simulink model "adcs_sim_main"  (R2016b)
settings: Solver=VariableStepAuto  StartTime=0.0  StopTime=360  RelTol=1e-3  EnableMultiTasking=on
InitFcn:
  | %sim_init
StopFcn:
  | %% Extract States
  | %states = logsout.getElement('states').Values;
  | %sc_quat = states.quaternion;
  | %omega_radps = states.body_rates_radps;
  | %pos_eci_km = states.position_eci_km;
  | %vel_eci_kmps = states.velocity_eci_kmps;
  | 
  | %% Extract Actuator measurements
  | %act_meas = logsout.getElement('act_meas').Values;
  | 
  | %% Extract Commands
  | %cmds = logsout.getElement('commands').Values;
  | %MT_dv = cmds.MT_dv;
  | 
  | %% Extract B-dot tumble status
  | %tumble = logsout.getElement('tumble').Values;
  | %tumble_t = logsout.getElement('tumble').Time;
undefined symbols (not defined in the file): adcs_fsw_main, CAN, CAN_lib, cmd_MT_fsw_dv, env_estimation_lib, Flightsoftware, fsw_params, MET, MSP_FSW, MSP_FSW_lib, orbit_TLE, sc_mode, sim_params
libraries: bus_stubs_fsw x2, actuators_lib x1, dynamics_lib x1, environment_lib x1, MET_lib x1, MSP_BDOT_lib x1, CAN_out_lib x1, extended_kalman_filter_lib x1, actuator_processing x1, command_generation x1, time_conversion_lib x1, gs_prediction_lib x1
settings Model: Creator=bbarz_000  LastModifiedBy=taylorreynolds
settings DataIOCC: SaveOutput=off
settings OptimizationCC: DefaultParameterBehavior=Inlined  UseDivisionForNetSlopeComputation=on  UseFloatMulNetSlope=on  InlineInvariantSignals=on  PassReuseOutputArgsAs=Individual arguments  ZeroExternalMemoryAtStartup=off  ZeroInternalMemoryAtStartup=off  NoFixptDivByZeroProtection=on  EfficientFloat2IntCast=on  LifeSpan=1
settings DebuggingCC: ParameterTunabilityLossMsg=error  SFUnexpectedBacktrackingDiag=warning  SFNoUnconditionalDefaultTransitionDiag=warning  SFExecutionAtInitializationDiag=none
settings HardwareCC: ProdBitPerInt=16  ProdBitPerPointer=16  ProdBitPerSizeT=16  ProdBitPerPtrDiffT=16  ProdLargestAtomicFloat=None  ProdWordSize=16  ProdHWDeviceType=Texas Instruments->MSP430
settings RTWCC: SystemTargetFile=ert.tlc  GenCodeOnly=on  PackageGeneratedCodeAndArtifacts=on  TemplateMakefile=ert_default_tmf  Description=Embedded Coder  GenerateReport=on  Toolchain=Clang v3.1 | gmake (64-bit Mac)  IncludeHyperlinkInReport=on  LaunchReport=on  GenerateTraceInfo=on  GenerateTraceReport=on  GenerateTraceReportSl=on  GenerateTraceReportSf=on  GenerateTraceReportEml=on  GenerateCodeMetricsReport=on
settings CodeAppCC: ForceParamTrailComments=on  IgnoreCustomStorageClasses=off  OperatorAnnotations=on  SimulinkDataObjDesc=on  SFDataObjDesc=on  MATLABFcnDesc=on  CustomSymbolStrGlobalVar=rt$N$M  CustomSymbolStrType=$N$M  CustomSymbolStrFcn=$N$M$F  CustomSymbolStrMacro=$N$M  InsertBlockDesc=on  MATLABSourceComments=on
settings ERTTargetCC: GenerateSampleERTMain=on  CombineSignalStateStructs=on  SupportComplex=off  SupportContinuousTime=on  SupportNonInlinedSFcns=on  InlinedParameterPlacement=NonHierarchical  ERTCustomFileTemplate=example_file_process.tlc  ERTFilePackagingFormat=CompactWithDataFile
settings ConfigComp: CovMetricSettings=dw  CovHtmlReporting=on  CovSaveCumulativeToWorkspaceVar=on  CovSaveSingleToWorkspaceVar=on  CovExternalEMLEnable=off

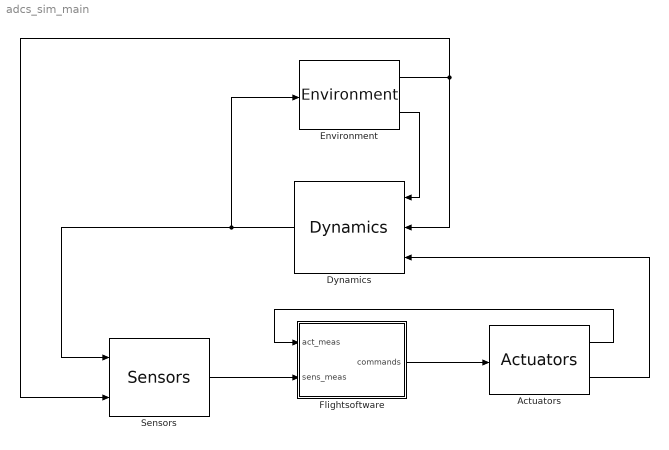
== system adcs_sim_main ==
  Actuators : actuators_lib/Actuators
  Dynamics : dynamics_lib/Dynamics
  Environment : environment_lib/Environment
  Flightsoftware : Subsystem  AncestorBlock=adcs_fsw_main/Flightsoftware
  Sensors : sensors_lib/Sensors
  wires:
  Flightsoftware/1(commands) -> Actuators/1
  Dynamics/1 -> Environment/1, Sensors/1
  Sensors/1 -> Flightsoftware/2(sens_meas)
  Environment/1 -> Sensors/2, Dynamics/2
  Actuators/2 -> Dynamics/3
  Actuators/1 -> Flightsoftware/1(act_meas)
  Environment/2 -> Dynamics/1

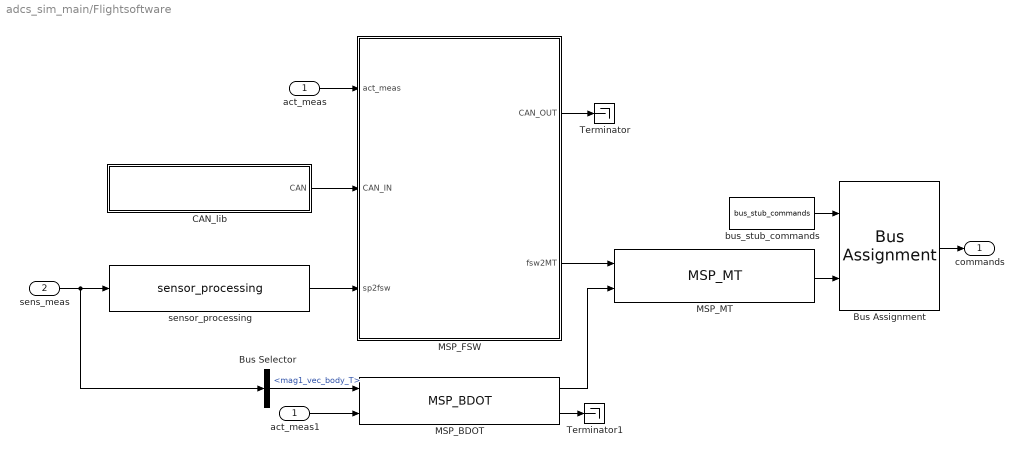
== system adcs_sim_main/Flightsoftware ==
  act_meas : Inport  OutDataTypeStr=Bus: act_meas
  sens_meas : Inport  Port=2  OutDataTypeStr=Bus: sens_meas
  Bus Assignment : BusAssignment  AssignedSignals=MT_dv
  Bus Selector : BusSelector  OutputSignals=mag1_vec_body_T
  CAN_lib : Subsystem  AncestorBlock=CAN_lib/CAN_lib
  MSP_BDOT : MSP_BDOT_lib/MSP_BDOT
  MSP_FSW : Subsystem  AncestorBlock=MSP_FSW_lib/MSP_FSW
  MSP_MT : MSP_MT_lib/MSP_MT
  Terminator : Terminator
  Terminator1 : Terminator
  act_meas1 : InportShadow  OutDataTypeStr=Bus: act_meas
  bus_stub_commands : bus_stubs_template/bus_stub_commands
  sensor_processing : sensor_processing/sensor_processing
  commands : Outport
  wires:
  act_meas1/1 -> MSP_BDOT/2
  MSP_BDOT/2 -> Terminator1/1
  MSP_FSW/1(CAN_OUT) -> Terminator/1
  CAN_lib/1(CAN) -> MSP_FSW/2(CAN_IN)
  act_meas/1 -> MSP_FSW/1(act_meas)
  sensor_processing/1 -> MSP_FSW/3(sp2fsw)
  MSP_FSW/2(fsw2MT) -> MSP_MT/1
  MSP_BDOT/1 -> MSP_MT/2
  MSP_MT/1 -> Bus Assignment/2
  Bus Selector/1 -> MSP_BDOT/1  "<mag1_vec_body_T>"
  sens_meas/1 -> Bus Selector/1, sensor_processing/1
  bus_stub_commands/1 -> Bus Assignment/1
  Bus Assignment/1 -> commands/1

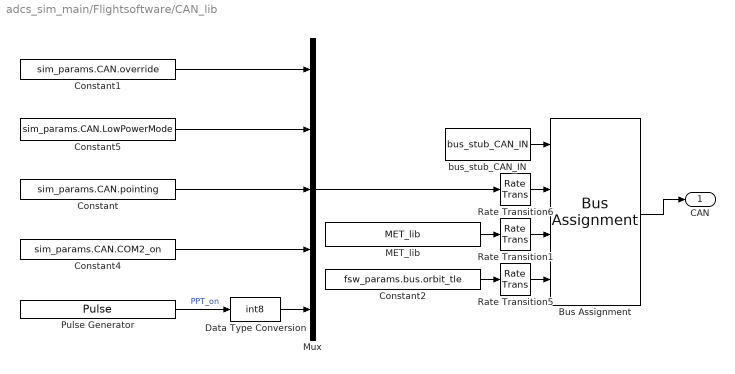
== system adcs_sim_main/Flightsoftware/CAN_lib ==
  Bus Assignment : BusAssignment  AssignedSignals=CAN,MET,orbit_TLE
  Constant : Constant  Value=sim_params.CAN.pointing  OutDataTypeStr=int8
  Constant1 : Constant  Value=sim_params.CAN.override  OutDataTypeStr=int8
  Constant2 : Constant  Value=fsw_params.bus.orbit_tle
  Constant4 : Constant  Value=sim_params.CAN.COM2_on  OutDataTypeStr=int8
  Constant5 : Constant  Value=sim_params.CAN.LowPowerMode  OutDataTypeStr=int8
  Data Type Conversion : DataTypeConversion  OutDataTypeStr=int8
  MET_lib : MET_lib/MET_lib
  Mux : Mux  Inputs=5
  Pulse Generator : DiscretePulseGenerator  PulseType=Time based  Period=sim_params.CAN.sync_pulse_period_s  PulseWidth=sim_params.CAN.PPT_on_sync_pct
  Rate Transition1 : RateTransition  X0=sim_params.CAN.ic.MET  OutPortSampleTime=sim_params.CAN.sample_time_s
  Rate Transition5 : RateTransition  X0=fsw_params.bus.orbit_tle  OutPortSampleTime=sim_params.CAN.sample_time_s
  Rate Transition6 : RateTransition  X0=sim_params.CAN.ic.all  OutPortSampleTime=sim_params.CAN.sample_time_s
  bus_stub_CAN_IN : bus_stubs_fsw/bus_stub_CAN_IN
  CAN : Outport
  wires:
  Data Type Conversion/1 -> Mux/5
  Rate Transition1/1 -> Bus Assignment/3
  Rate Transition6/1 -> Bus Assignment/2
  Rate Transition5/1 -> Bus Assignment/4
  Constant2/1 -> Rate Transition5/1
  MET_lib/1 -> Rate Transition1/1
  Pulse Generator/1 -> Data Type Conversion/1  "PPT_on"
  Constant4/1 -> Mux/4
  Constant/1 -> Mux/3
  Constant5/1 -> Mux/2
  Constant1/1 -> Mux/1
  Mux/1 -> Rate Transition6/1
  bus_stub_CAN_IN/1 -> Bus Assignment/1
  Bus Assignment/1 -> CAN/1

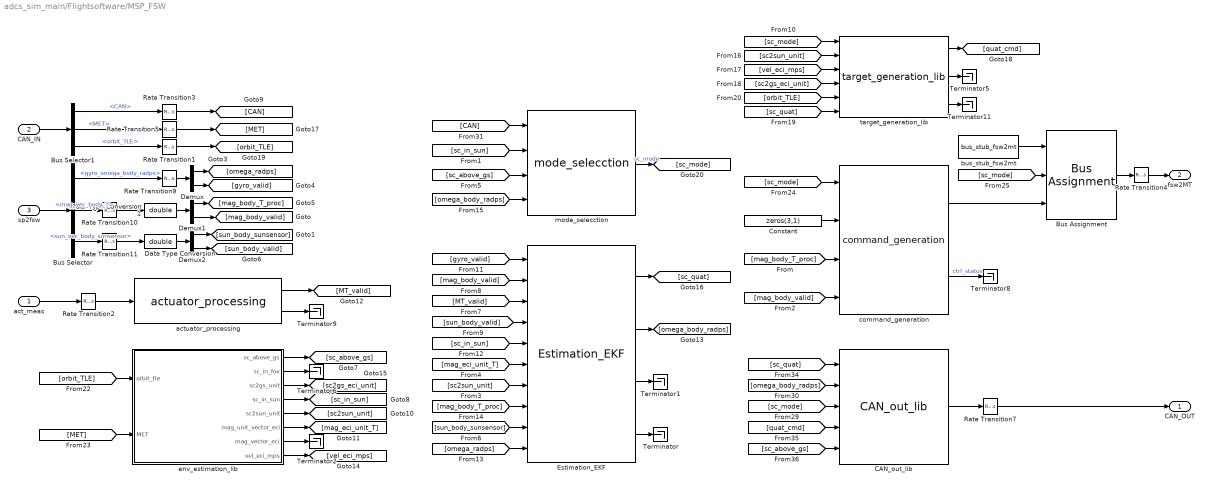
== system adcs_sim_main/Flightsoftware/MSP_FSW ==
  act_meas : Inport
  CAN_IN : Inport  Port=2  OutDataTypeStr=Bus: CAN_IN
  sp2fsw : Inport  Port=3  OutDataTypeStr=Bus: sp2fsw
  Bus Assignment : BusAssignment  AssignedSignals=sc_mode,cmd_MT_fsw_dv
  Bus Selector : BusSelector  OutputSignals=gyro_omega_body_radps,mag_vec_body_T,sun_vec_body_sunsensor
  Bus Selector1 : BusSelector  OutputSignals=CAN,MET,orbit_TLE
  CAN_out_lib : CAN_out_lib/CAN_out_lib
  Constant : Constant  Value=zeros(3,1)
  Data Type Conversion : DataTypeConversion  OutDataTypeStr=double
  Data Type Conversion1 : DataTypeConversion  OutDataTypeStr=double
  Demux : Demux  Outputs=[3 1]
  Demux1 : Demux  Outputs=[3 1]
  Demux2 : Demux  Outputs=[3 1]
  "Estimation_EKF " : extended_kalman_filter_lib/Estimation_EKF 
  Rate Transition1 : RateTransition  X0=fsw_params.bus.orbit_tle  OutPortSampleTime=fsw_params.sample_time_s
  Rate Transition{2,9..11} (4 alike) : RateTransition  OutPortSampleTime=fsw_params.sample_time_s
  Rate Transition3 : RateTransition  X0=fsw_params.bus.CAN_ic  OutPortSampleTime=fsw_params.sample_time_s
  Rate Transition4 : RateTransition
  Rate Transition5 : RateTransition  X0=fsw_params.bus.MET_epoch  OutPortSampleTime=fsw_params.sample_time_s
  Rate Transition7 : RateTransition
  Terminator{,1..2,5..6,8..9,11} (8 alike) : Terminator
  actuator_processing : actuator_processing/actuator_processing
  bus_stub_fsw2mt : bus_stubs_fsw/bus_stub_fsw2mt
  command_generation : command_generation/command_generation
  env_estimation_lib : Subsystem  AncestorBlock=env_estimation_lib/env_estimation_lib
  mode_selecction : mode_selection/mode_selecction
  target_generation_lib : target_generation_lib/target_generation_lib
  CAN_OUT : Outport
  fsw2MT : Outport  Port=2
  wires:
  Data Type Conversion1/1 -> Demux1/1
  Data Type Conversion/1 -> Demux2/1
  Demux1/2 -> [mag_body_valid]
  Demux1/1 -> [mag_body_T_proc]
  Bus Selector1/2 -> Rate Transition5/1  "<MET>"
  Rate Transition5/1 -> [MET]
  [sc_mode] -> Bus Assignment/2
  [sc_mode] -> command_generation/1
  [sc_mode] -> target_generation_lib/1
  mode_selecction/1 -> [sc_mode]  "sc_mode"
  [MET] -> env_estimation_lib/2(MET)
  [orbit_TLE] -> env_estimation_lib/1(orbit_tle)
  Bus Selector1/3 -> Rate Transition1/1  "<orbit_TLE>"
  Rate Transition1/1 -> [orbit_TLE]
  Constant/1 -> command_generation/2
  command_generation/1 -> Bus Assignment/3
  [mag_body_T_proc] -> command_generation/3
  [quat_cmd] -> CAN_out_lib/4
  target_generation_lib/3 -> Terminator11/1
  [sc_above_gs] -> CAN_out_lib/5
  [sc_quat] -> CAN_out_lib/1
  [omega_body_radps] -> CAN_out_lib/2
  [sc_mode] -> CAN_out_lib/3
  [CAN] -> mode_selecction/1
  Rate Transition7/1 -> CAN_OUT/1
  Rate Transition4/1 -> fsw2MT/1
  CAN_IN/1 -> Bus Selector1/1
  Rate Transition2/1 -> actuator_processing/1
  sp2fsw/1 -> Bus Selector/1
  CAN_out_lib/1 -> Rate Transition7/1
  Bus Assignment/1 -> Rate Transition4/1
  bus_stub_fsw2mt/1 -> Bus Assignment/1
  target_generation_lib/2 -> Terminator5/1
  target_generation_lib/1 -> [quat_cmd]
  [orbit_TLE] -> target_generation_lib/5
  [sc_quat] -> target_generation_lib/6
  [sc2gs_eci_unit] -> target_generation_lib/4
  [vel_eci_mps] -> target_generation_lib/3
  [sc2sun_unit] -> target_generation_lib/2
  [omega_body_radps] -> mode_selecction/4
  "Estimation_EKF "/2 -> [omega_body_radps]
  actuator_processing/2 -> Terminator9/1
  actuator_processing/1 -> [MT_valid]
  act_meas/1 -> Rate Transition2/1
  Demux2/2 -> [sun_body_valid]
  Demux2/1 -> [sun_body_sunsensor]
  Bus Selector/3 -> Rate Transition11/1  "<sun_vec_body_sunsensor>"
  Rate Transition10/1 -> Data Type Conversion1/1
  Bus Selector/2 -> Rate Transition10/1  "<mag_vec_body_T>"
  Demux/2 -> [gyro_valid]
  Demux/1 -> [omega_radps]
  Bus Selector/1 -> Rate Transition9/1  "<gyro_omega_body_radps>"
  [sc_in_sun] -> mode_selecction/2
  [mag_body_valid] -> "Estimation_EKF "/2
  [gyro_valid] -> "Estimation_EKF "/1
  env_estimation_lib/4(sc_in_sun) -> [sc_in_sun]
  [MT_valid] -> "Estimation_EKF "/3
  [sun_body_valid] -> "Estimation_EKF "/4
  [sc_in_sun] -> "Estimation_EKF "/5
  "Estimation_EKF "/4 -> Terminator/1
  "Estimation_EKF "/3 -> Terminator1/1
  env_estimation_lib/5(sc2sun_unit) -> [sc2sun_unit]
  env_estimation_lib/6(mag_unit_vector_eci) -> [mag_eci_unit_T]
  env_estimation_lib/7(mag_vector_eci) -> Terminator2/1
  env_estimation_lib/8(vel_eci_mps) -> [vel_eci_mps]
  env_estimation_lib/2(sc_in_fov) -> Terminator6/1
  env_estimation_lib/3(sc2gs_unit) -> [sc2gs_eci_unit]
  [omega_radps] -> "Estimation_EKF "/10
  [sun_body_sunsensor] -> "Estimation_EKF "/9
  [mag_body_T_proc] -> "Estimation_EKF "/8
  [mag_eci_unit_T] -> "Estimation_EKF "/6
  [sc2sun_unit] -> "Estimation_EKF "/7
  [mag_body_valid] -> command_generation/4
  command_generation/2 -> Terminator8/1  "ctrl_status"
  "Estimation_EKF "/1 -> [sc_quat]
  env_estimation_lib/1(sc_above_gs) -> [sc_above_gs]
  [sc_above_gs] -> mode_selecction/3
  Rate Transition9/1 -> Demux/1
  Rate Transition11/1 -> Data Type Conversion/1
  Bus Selector1/1 -> Rate Transition3/1  "<CAN>"
  Rate Transition3/1 -> [CAN]

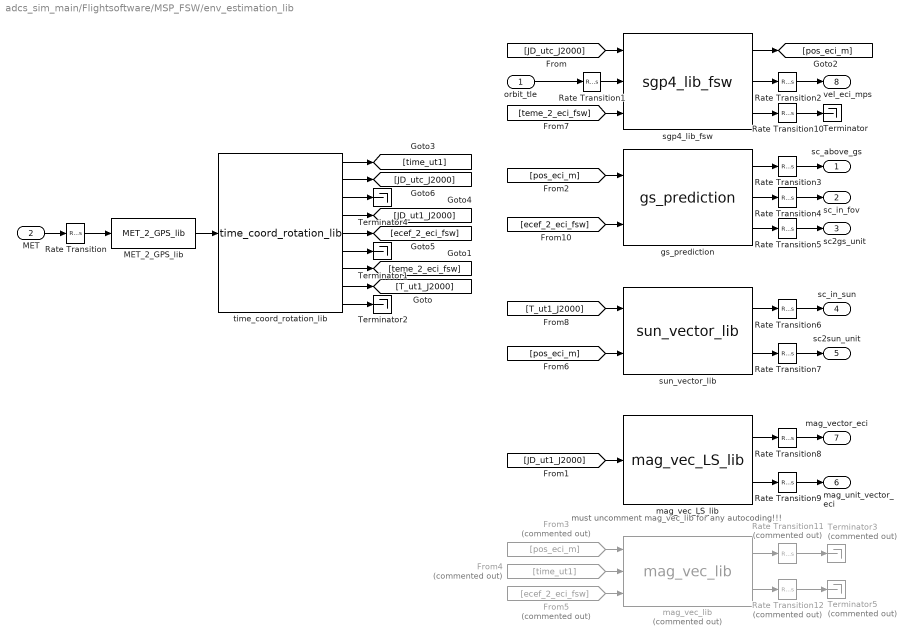
== system adcs_sim_main/Flightsoftware/MSP_FSW/env_estimation_lib ==
  note: must uncomment mag_vec_lib for any autocoding!!!
  orbit_tle : Inport
  MET : Inport  Port=2
  From3 : From  Commented=on  GotoTag=pos_eci_m
  From4 : From  Commented=on  GotoTag=time_ut1
  From5 : From  Commented=on  GotoTag=ecef_2_eci_fsw
  MET_2_GPS_lib : time_conversion_lib/MET_2_GPS_lib
  Rate Transition : RateTransition  X0=fsw_params.constants.ic.time.JD_J2000_TT_s  OutPortSampleTime=fsw_params.env_estimation.sample_time_s
  Rate Transition1 : RateTransition  X0=fsw_params.env_estimation.ic.orbit_tle  OutPortSampleTime=fsw_params.env_estimation.sample_time_s
  Rate Transition{2..10} (9 alike) : RateTransition
  Rate Transition11 : RateTransition  Commented=on
  Rate Transition12 : RateTransition  Commented=on
  Terminator{,1..2,4} (4 alike) : Terminator
  Terminator3 : Terminator  Commented=on
  Terminator5 : Terminator  Commented=on
  gs_prediction : gs_prediction_lib/gs_prediction
  mag_vec_LS_lib : mag_vec_LS_lib/mag_vec_LS_lib
  mag_vec_lib : mag_vec_lib/mag_vec_lib  Commented=on
  sgp4_lib_fsw : sgp4_lib_fsw/sgp4_lib_fsw
  sun_vector_lib : sun_vector_lib/sun_vector_lib
  time_coord_rotation_lib : time_coord_rotation_lib/time_coord_rotation_lib
  sc_above_gs : Outport
  sc_in_fov : Outport  Port=2
  sc2gs_unit : Outport  Port=3
  sc_in_sun : Outport  Port=4
  sc2sun_unit : Outport  Port=5
  mag_unit_vector_eci : Outport  Port=6
  mag_vector_eci : Outport  Port=7
  vel_eci_mps : Outport  Port=8
  wires:
  Rate Transition12/1 -> Terminator5/1
  Rate Transition11/1 -> Terminator3/1
  From5/1 -> mag_vec_lib/3
  From4/1 -> mag_vec_lib/2
  From3/1 -> mag_vec_lib/1
  mag_vec_lib/2 -> Rate Transition12/1
  mag_vec_lib/1 -> Rate Transition11/1
  [JD_ut1_J2000] -> mag_vec_LS_lib/1
  MET_2_GPS_lib/1 -> time_coord_rotation_lib/1
  Rate Transition/1 -> MET_2_GPS_lib/1
  Rate Transition10/1 -> Terminator/1
  sgp4_lib_fsw/3 -> Rate Transition10/1
  sgp4_lib_fsw/2 -> Rate Transition2/1
  [teme_2_eci_fsw] -> sgp4_lib_fsw/3
  time_coord_rotation_lib/2 -> [JD_utc_J2000]
  time_coord_rotation_lib/3 -> Terminator4/1
  time_coord_rotation_lib/4 -> [JD_ut1_J2000]
  time_coord_rotation_lib/5 -> [ecef_2_eci_fsw]
  time_coord_rotation_lib/6 -> Terminator1/1
  time_coord_rotation_lib/7 -> [teme_2_eci_fsw]
  time_coord_rotation_lib/8 -> [T_ut1_J2000]
  time_coord_rotation_lib/9 -> Terminator2/1
  [pos_eci_m] -> gs_prediction/1
  [ecef_2_eci_fsw] -> gs_prediction/2
  Rate Transition9/1 -> mag_unit_vector_eci/1
  Rate Transition8/1 -> mag_vector_eci/1
  Rate Transition7/1 -> sc2sun_unit/1
  Rate Transition6/1 -> sc_in_sun/1
  Rate Transition5/1 -> sc2gs_unit/1
  Rate Transition4/1 -> sc_in_fov/1
  Rate Transition3/1 -> sc_above_gs/1
  Rate Transition2/1 -> vel_eci_mps/1
  Rate Transition1/1 -> sgp4_lib_fsw/2
  gs_prediction/2 -> Rate Transition4/1
  gs_prediction/3 -> Rate Transition5/1
  gs_prediction/1 -> Rate Transition3/1
  time_coord_rotation_lib/1 -> [time_ut1]
  MET/1 -> Rate Transition/1
  orbit_tle/1 -> Rate Transition1/1
  sgp4_lib_fsw/1 -> [pos_eci_m]
  [pos_eci_m] -> sun_vector_lib/2
  sun_vector_lib/1 -> Rate Transition6/1
  [JD_utc_J2000] -> sgp4_lib_fsw/1
  [T_ut1_J2000] -> sun_vector_lib/1
  sun_vector_lib/2 -> Rate Transition7/1
  mag_vec_LS_lib/1 -> Rate Transition8/1
  mag_vec_LS_lib/2 -> Rate Transition9/1
